simulink model "Simplified_PMSM_Vehicle"  (R2024a)
settings: Solver=ode15s  StartTime=0.0  StopTime=10  RelTol=1e-3  AbsTol=1e-3
undefined symbols (not defined in the file): A, Ca, Ff, Fg, p
libraries: fl_lib x35, nesl_utility x15, ee_lib x3, batteryecm_lib x1
settings Model: Creator=macbookair  LastModifiedBy=macbookair
settings SolverCC: AutoScaleAbsTol=off  AlgebraicLoopSolver=TrustRegion  MaxZcPerStep=1
settings DebuggingCC: UnconnectedInputMsg=warning  UnconnectedOutputMsg=warning  UnconnectedLineMsg=warning  SymbolicDimsDataTypeCodeGenerationDiagnostic=none
settings ModelReferenceCC: EnableRefExpFcnMdlSchedulingChecks=on
settings SFSimCC: CustomCodeUndefinedFunction=UseInterfaceOnly
settings RTWCC: GPUComputeCapability=3.5  DLArmComputeVersion=19.05
settings SimscapeCC: SimscapeLogType=all  SimscapeLogSimulationStatistics=on  SimscapeLogDataHistory=10000

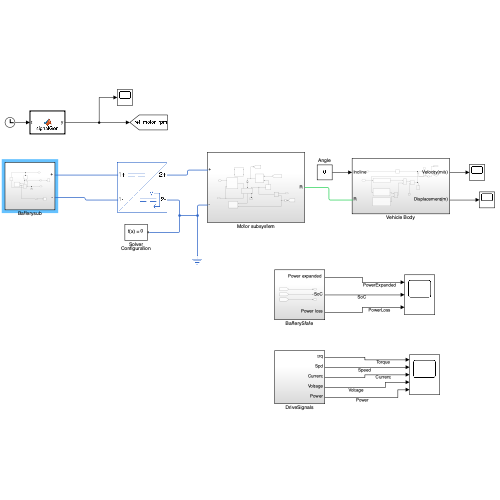
[thumbnail: Simulink's stored preview of the top-level diagram]
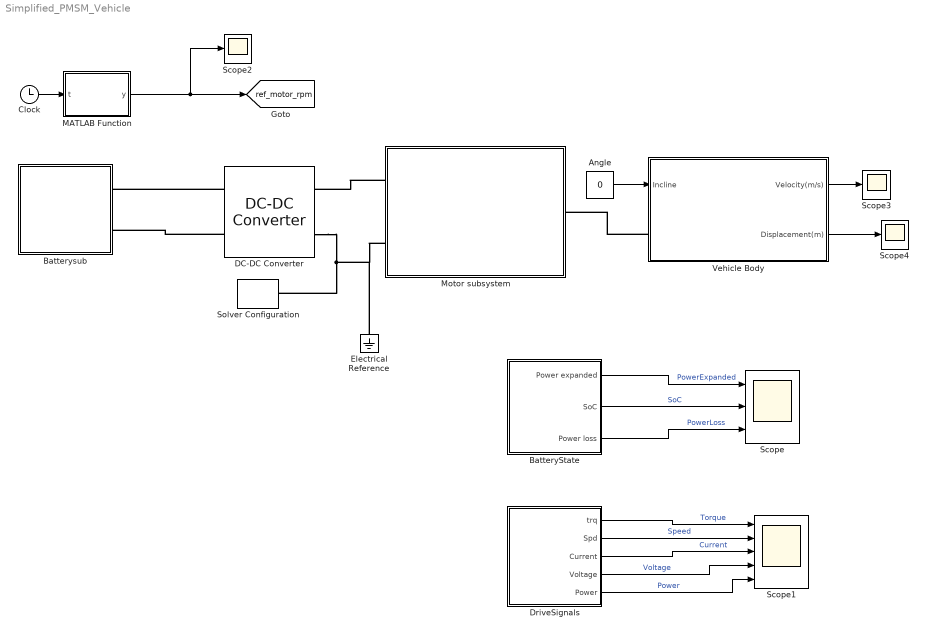
== system Simplified_PMSM_Vehicle ==
  Angle : Constant  Value=0
  BatteryState : Subsystem
  Batterysub : Subsystem
  Clock : Clock
  DC-DC Converter : ee_lib/Semiconductors & Converters/Converters/DC-DC Converter  Vref_option=ee.enum.converters.voltageref.internal  v_ref=500 V  P_rated=200 kW  droop_enabled=true  droop_param=ee.enum.converters.droop.value  droop=0.1 V/A  droop_percent=2  Vref_droop=10 V  reversible=ee.enum.converters.directionality.bidirectional  G_diode=1e-8 1/Ohm  P_fixed=100 W  losses_option=ee.enum.converters.lossesOption.proportionalToSquaredCurrent  eff_rated=97  tableOption=ee.enum.converters.lossTableOptionThermal.currentTemp  i_eff_vec=[-2, -1, 1, 2] A  v_eff_vec=[15, 30, 45] V  eff_vec=[66, 76, 80, 74]  eff_2D_table=[66, 66, 66; 76, 76, 76; 80, 80, 80; 74, 74, 74]  model_dynamics=ee.enum.converters.dynamics.yes  tau=0.02 s  v_ini=500 V  v1_min=1 V  R1=1000 Ohm  R2=1000 Ohm  enable_fault=simscape.enum.onoff.off  fault_condition=ee.enum.faults.faultInputCondition.greaterThan  fault_threshold=0.5  T_eff_vec=[280, 300, 320] K  eff_3D_table=repmat([66; 76; 80; 74], 1, 3, 3)  thermal_mass=100 J/K  initial_temperature=298.15 K
      settings: InternalSimscapePortConfiguration="{\"Bottom\":[],\"Left\":[{\"id\":\"p1\",\"label\":\"1+\",\"type\":\"foundation.electrical.electrical\"},{\"id\":\"n1\",\"label\":\"1-\",\"type\":\"foundation.electrical.electrical\"}],\"Right\":[{\"id\":\"p2\",\"label\":\"2+\",\"type\":\"foundation.electrical.electrical\"},{\"id\":\"n2\",\"label\":\"2-\",\"type\":\"foundation.electrical.electrical\"}],\"Top\":[]}"
  DriveSignals : Subsystem
  Electrical Reference : fl_lib/Electrical/Electrical Elements/Electrical Reference
  MATLAB Function : MATLAB Function  TreatAsAtomicUnit=on
  Motor subsystem : Subsystem
  Scope : Scope  NumInputPorts=3
  Scope1 : Scope  NumInputPorts=5
  Scope2 : Scope
  Scope3 : Scope
  Scope4 : Scope
  Solver Configuration : nesl_utility/Solver Configuration  PhysicalDomain=network_engine_domain  SubClassName=solver  LeftPortType=input  RightPortType=generic  Tones=[]  Harmonics=[]  SimulateNoise=off  Profile=off  UseLocalSampling=off  EnableSwitchedLinearOptims=on  FrequencyDomain=off  UseCCode=off  RelTol=0.001  AbsTol=1e-06  MinStep=1e-09  ToWorkspace=off  RevertToSquareIcSolve=off  NumHomotopyIterations=100  PhasorMode=off  PhasorModeNumHarmonics=1  ConsistencySolver=NEWTON_XTOL_AFTER_FTOL  IndexReductionMethod=DerivativeReplacement  DoDC=off  ResidualTolerance=1e-09  ConsistencyTolSource=GLOBAL  ConsistencyAbsTol=0.001  ConsistencyRelTol=0.001  ConsistencyTolFactor=0.001  UseLocalSolver=off  LocalSolverChoice=NE_BACKWARD_EULER_ADVANCER  ResolveIndetEquations=on  FunctionEvalNumThread=1  LocalSolverSampleTime=0.001  DoFixedCost=off  MaxNonlinIter=3  MaxModeIter=2  ComputeImpulses=off  ImpulseIterations=2  LinearAlgebra=auto  LinearAlgebraNumThread=0  EquationFormulation=NE_TIME_EF  DelaysMemoryBudget=1024  AutomaticFiltering=on  FilteringTimeConstant=0.001  PartitionStorageMethod=AS_NEEDED  PartitionMemoryBudget=1024  PartitionMethod=ROBUST  MultibodyUseLocalSolver=off  MultibodyLocalSolverChoice=ODE1  MultibodyLocalSolverSampleTime=0.001
  Vehicle Body : Subsystem
  tag scope: ref_motor_rpm=global
  wires:
  Clock/1 -> MATLAB Function/1(t)
  Angle/1 -> Vehicle Body/1(Incline)
  BatteryState/1("Power expanded ") -> Scope/1  "PowerExpanded"
  BatteryState/2(SoC) -> Scope/2  "SoC"
  BatteryState/3(Power loss) -> Scope/3  "PowerLoss"
  DriveSignals/1(trq) -> Scope1/1  "Torque"
  DriveSignals/2(Spd) -> Scope1/2  "Speed"
  DriveSignals/3(Current) -> Scope1/3  "Current"
  DriveSignals/4(Voltage) -> Scope1/4  "Voltage"
  DriveSignals/5(Power) -> Scope1/5  "Power"
  MATLAB Function/1(y) -> Scope2/1, [ref_motor_rpm]
  Vehicle Body/1(Velocity(m/s)) -> Scope3/1
  Vehicle Body/2(Displacement(m)) -> Scope4/1
  connections:
  DC-DC Converter/LConn1 -- Batterysub/LConn1
  DC-DC Converter/LConn2 -- Batterysub/LConn2
  DC-DC Converter/RConn2 -- Motor subsystem/LConn2 -- Electrical Reference/LConn1 -- Solver Configuration/RConn1
  Vehicle Body/LConn1 -- Motor subsystem/RConn1
  Motor subsystem/LConn1 -- DC-DC Converter/RConn1

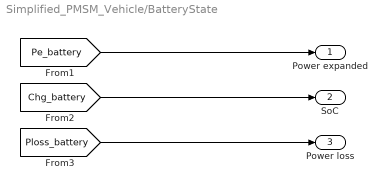
== system Simplified_PMSM_Vehicle/BatteryState ==
  "Power expanded " : Outport
  SoC : Outport  Port=2
  Power loss : Outport  Port=3
  wires:
  [Pe_battery] -> "Power expanded "/1
  [Chg_battery] -> SoC/1
  [Ploss_battery] -> Power loss/1

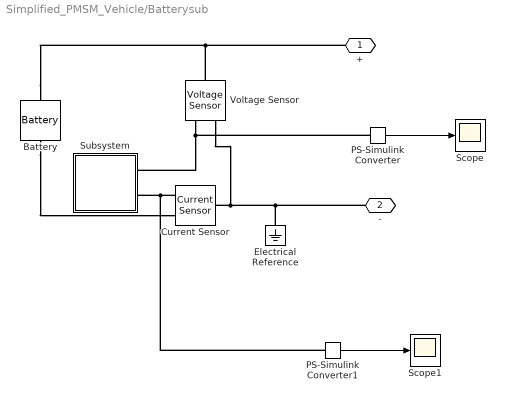
== system Simplified_PMSM_Vehicle/Batterysub ==
  Battery : batteryecm_lib/Battery  Vnom=201.6 V  prm_dir=simscape.enum.battery.prm_dir.disabled  R1_dis=2 Ohm  R1_ch=2 Ohm  R1=0.05 Ohm  prm_AH=simscape.enum.battery.prm_AH.finite  AH=150 A*hr  V1=190 V  AH1=75 A*hr  prm_R2=simscape.enum.battery.prm_R2.disabled  R2=2000 Ohm  Tmeas=298.15 K  charge_measurement_port=simscape.enum.battery.enable.no  prm_dyn=simscape.enum.battery.prm_dyn.off  Rp1=0.005 Ohm  tau1=30 s  Rp2=0.005 Ohm  tau2=30 s  Rp3=0.005 Ohm  tau3=30 s  Rp4=0.005 Ohm  tau4=30 s  Rp5=0.005 Ohm  tau5=30 s  prm_fade=simscape.enum.battery.prm_fade.disabled  N_fade=100  AH_fade=45 A*hr  R1_fade=2.02 Ohm  R1_ch_fade=2.02 Ohm  V1_fade=10.35 V  prm_age=simscape.enum.battery.prm_age.disabled  prm_age_OCV=simscape.enum.battery.prm_age_OCV.OCV  OCV_age=0.9  SOC_age=60  Tmeas_age=298.15 K  delta_time_age_vec=[0] d  temperature_age_vec=[273] K  OCV_scaling_age=2.2134e6  OCV_offset_age=1.632e6  temp_exp_age=0.515833569 V  t_exp_age=0.75  Vnom_T2=12 V  R1_T2=2.2 Ohm  R1_T2_dis=2.2 Ohm  R1_T2_ch=2.2 Ohm  V1_T2=11.4 V  R2_T2=2200 Ohm  Rp1_T2=0.005 Ohm  tau1_T2=30 s  Rp2_T2=0.005 Ohm  tau2_T2=30 s  Rp3_T2=0.005 Ohm  tau3_T2=30 s  Rp4_T2=0.005 Ohm  tau4_T2=30 s  Rp5_T2=0.005 Ohm  tau5_T2=30 s  Tmeas2=273.15 K  thermal_port=simscape.enum.thermaleffects.omit  thermal_mass=30000 J/K  i_specify=off  i_priority=None  i=0 A  i_nominal_specify=off  i_nominal_value=1  i_nominal_unit=A  v_specify=off  v_priority=None  v=0 V  v_nominal_specify=off  v_nominal_value=1  v_nominal_unit=V  charge_specify=on  charge_priority=High  charge=100 A*hr  charge_nominal_specify=off  charge_nominal_value=1  charge_nominal_unit=A*hr  num_cycles_specify=off  num_cycles_priority=High  num_cycles=0  num_cycles_nominal_specify=off  num_cycles_nominal_value=1  num_cycles_nominal_unit=1  temperature_specify=off  temperature_priority=High  temperature=298.15 K  temperature_nominal_specify=off  temperature_nominal_value=1  temperature_nominal_unit=K
  Current Sensor : fl_lib/Electrical/Electrical Sensors/Current Sensor
  Electrical Reference : fl_lib/Electrical/Electrical Elements/Electrical Reference
  PS-Simulink Converter : nesl_utility/PS-Simulink Converter  PhysicalDomain=network_engine_domain  SubClassName=ps_output  LeftPortType=input  RightPortType=output  PseudoPeriodic=off  Frequencies=[]  VectorFormat=inherit  Unit=inherit  AffineConversion=off
  PS-Simulink Converter1 : nesl_utility/PS-Simulink Converter  PhysicalDomain=network_engine_domain  SubClassName=ps_output  LeftPortType=input  RightPortType=output  PseudoPeriodic=off  Frequencies=[]  VectorFormat=inherit  Unit=inherit  AffineConversion=off
  Scope : Scope
  Scope1 : Scope
  Subsystem : Subsystem
  Voltage Sensor : fl_lib/Electrical/Electrical Sensors/Voltage Sensor
  + : PMIOPort  Side=Left
  - : PMIOPort  Port=2  Side=Left
  wires:
  PS-Simulink Converter/1 -> Scope/1
  PS-Simulink Converter1/1 -> Scope1/1
  connections:
  Current Sensor/RConn1 -- PS-Simulink Converter1/LConn1 -- Subsystem/LConn2
  Battery/LConn1 -- +/RConn1 -- Voltage Sensor/LConn1
  Electrical Reference/LConn1 -- -/RConn1 -- Voltage Sensor/RConn2 -- Current Sensor/LConn1
  Voltage Sensor/RConn1 -- Subsystem/LConn1 -- PS-Simulink Converter/LConn1
  Battery/RConn1 -- Current Sensor/RConn2

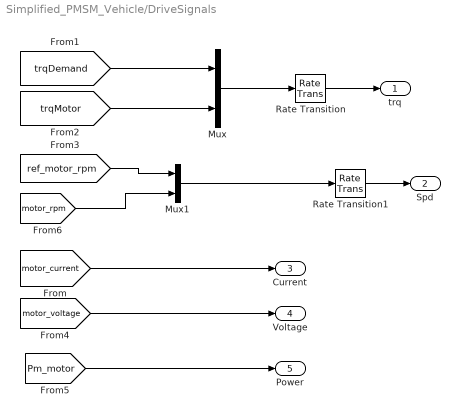
== system Simplified_PMSM_Vehicle/DriveSignals ==
  Mux : Mux  Inputs=2
  Mux1 : Mux  Inputs=2
  Rate Transition : RateTransition
  Rate Transition1 : RateTransition
  trq : Outport
  Spd : Outport  Port=2
  Current : Outport  Port=3
  Voltage : Outport  Port=4
  Power : Outport  Port=5
  wires:
  [trqDemand] -> Mux/1
  [trqMotor] -> Mux/2
  [ref_motor_rpm] -> Mux1/1
  [motor_rpm] -> Mux1/2
  Mux1/1 -> Rate Transition1/1
  Mux/1 -> Rate Transition/1
  [motor_current] -> Current/1
  [motor_voltage] -> Voltage/1
  [Pm_motor] -> Power/1
  Rate Transition/1 -> trq/1
  Rate Transition1/1 -> Spd/1

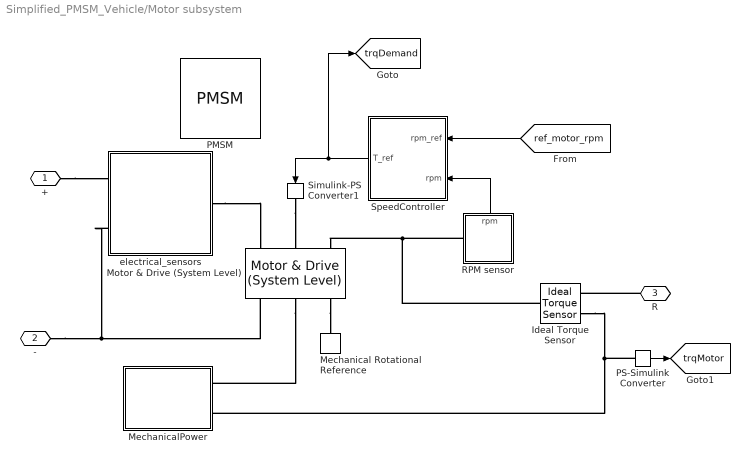
== system Simplified_PMSM_Vehicle/Motor subsystem ==
  Ideal Torque Sensor : fl_lib/Mechanical/Mechanical Sensors/Ideal Torque Sensor
  Mechanical Rotational Reference : fl_lib/Mechanical/Rotational Elements/Mechanical Rotational Reference
  MechanicalPower : Subsystem
  Motor & Drive (System Level) : ee_lib/Electromechanical/Motor & Drive (System Level)  torque_speed_param=ee.enum.electromech.envelope.tabulated  overtorque_param=ee.enum.electromech.overtorque.no  T_t=[.09, .08, .07, 0]*500 N*m  T_t_intermittent=[.36, .32, .28, 0] N*m  T_t_2D=[.09, .09, .09; .08, .08, .08; .07, .07, .07; 0, 0, 0] N*m  T_t_intermittent_2D=[.36, .36, .36; .32, .32, .32; .28, .28, .28; 0, 0, 0] N*m  w_t=[0, 3750, 7500, 8000] rpm  vdc_t=[6, 12, 24] V  torque_max=0.1 N*m  power_max=30 W  torque_max_intermittent=0.4 N*m  power_max_intermittent=120 W  time_overtorque=30 s  time_recover=60 s  Tc=0.02 s  EnableSwitch=false  losses_param=1  eff=95  w_eff=3750 rpm  T_eff=400 N*m  Piron=0 W  Pbase=0 W  w_eff_vec=[-8000, -4000, 0, 4000, 8000] rpm  T_eff_vec=[0, .03, .06, .09] N*m  v_eff_vec=[100, 250, 400] V  losses_mat=[1.49, 1.67, 2.21, 3.1; .42, .69, 1.14, 2.03; .06, .24, .78, 1.68; .42, .69, 1.14, 2.03; 1.49, 1.67, 2.21, 3.1] W  efficiency_mat=[95, 95, 95, 95; 95, 95, 95, 95; 95, 95, 95, 95; 95, 95, 95, 95; 95, 95, 95, 95]  losses_mat_3D=ones(5, 4, 3) W  efficiency_mat_3D=95 * ones(5, 4, 3)  Res=0 Ohm  enable_fault=simscape.enum.onoff.off  fault_condition=1  fault_threshold=0.5  J=0 kg*m^2  lam=1e-5 N*m*s/rad  speed0=0 rpm  faulted_specify=off  faulted_priority=None  faulted=0  faulted_nominal_specify=off  faulted_nominal_value=1  faulted_nominal_unit=1  isSwitchedOff_specify=off  isSwitchedOff_priority=None  isSwitchedOff=0  isSwitchedOff_nominal_specify=off  isSwitchedOff_nominal_value=1  isSwitchedOff_nominal_unit=1  torqueLimitContinuous_specify=off  torqueLimitContinuous_priority=None  torqueLimitContinuous=0 N*m  torqueLimitContinuous_nominal_specify=off  torqueLimitContinuous_nominal_value=1  torqueLimitContinuous_nominal_unit=N*m  alpha=3.93e-3 1/K  Tmeas=25 degC  Tmeas2=125 degC  losses_mat_T2=[1.49, 1.74, 2.49, 3.74; .42, .67, 1.42, 2.67; .06, .31, 1.06, 2.31; .42, .67, 1.42, 2.67; 1.49, 1.74, 2.49, 3.74] W  efficiency_mat_T2=[95, 95, 95, 95; 95, 95, 95, 95; 95, 95, 95, 95; 95, 95, 95, 95; 95, 95, 95, 95]  losses_mat_3D_T2=ones(5, 4, 3) W  efficiency_mat_3D_T2=95 * ones(5, 4, 3)  thermal_mass=100 J/K  initial_temperature=25 degC
  PMSM : ee_lib/Electromechanical/Permanent Magnet/PMSM  port_option=ee.enum.threePhasePort.composite  winding_type=ee.enum.electromech.statorconfiguration.wye  machine_param=ee.enum.pmsm.parameterization.constant  nPolePairs=6  pmflux_param=ee.enum.pmflux.fluxlinkage  pm_flux_linkage=0.03 Wb  torque_constant=0.18 N*m/A  back_emf_constant=0.18 V*s/rad  stator_param=ee.enum.statorparam.LdLqL0  Ld=0.00019 H  Lq=0.00025 H  idVec=[-200, 0, 200] A  iqVec=[-200, 0, 200] A  LdMatrix=0.0002 * ones(3, 3) H  LqMatrix=0.0002 * ones(3, 3) H  PmMatrix=0.1 * ones(3, 3) Wb  ktMatrix=0.18 * ones(3, 3) N*m/A  keMatrix=0.18 * ones(3, 3) V*s/rad  L0=0.00016 H  Ls=0.0002 H  Lm=-0.00002 H  Ms=0.00002 H  Rs=0.013 Ohm  zero_sequence=ee.enum.park.zerosequence.include  axes_param=ee.enum.rotorangle.daxis  loss_param=ee.enum.ironloss.none  losses_oc=[0, 0, 0] W  losses_sc=[0, 0, 0] W  f_losses=60 Hz  Isc_losses=95 A  J=0.01 kg*m^2  lam=0 N*m*s/rad  i_d_specify=off  i_d_priority=None  i_d=0 A  i_d_nominal_specify=off  i_d_nominal_value=1  i_d_nominal_unit=A  i_q_specify=off  i_q_priority=None  i_q=0 A  i_q_nominal_specify=off  i_q_nominal_value=1  i_q_nominal_unit=A  torque_specify=off  torque_priority=None  torque=0 N*m  torque_nominal_specify=off  torque_nominal_value=1  torque_nominal_unit=N*m  angular_velocity_specify=off  angular_velocity_priority=High  angular_velocity=0 rpm  angular_velocity_nominal_specify=off  angular_velocity_nominal_value=1  angular_velocity_nominal_unit=rpm  angular_position_specify=off  angular_position_priority=High  angular_position=0 deg  angular_position_nominal_specify=off  angular_position_nominal_value=1  angular_position_nominal_unit=deg  alpha=3.93e-3 1/K  alpha_flux=-0.001 1/K  Tmeas=298.15 K  stator_thermal_mass=100 J/K  rotor_thermal_mass=200 J/K  Rm_percent_rotor=90  Rd_percent_rotor=30  temperatureA_specify=off  temperatureA_priority=High  temperatureA=25 degC  temperatureA_nominal_specify=off  temperatureA_nominal_value=1  temperatureA_nominal_unit=degC  temperatureB_specify=off  temperatureB_priority=High  temperatureB=25 degC  temperatureB_nominal_specify=off  temperatureB_nominal_value=1  temperatureB_nominal_unit=degC  temperatureC_specify=off  temperatureC_priority=High  temperatureC=25 degC  temperatureC_nominal_specify=off  temperatureC_nominal_value=1  temperatureC_nominal_unit=degC  temperatureR_specify=off  temperatureR_priority=High  temperatureR=25 degC  temperatureR_nominal_specify=off  temperatureR_nominal_value=1  temperatureR_nominal_unit=degC
      settings: InternalSimscapePortConfiguration="{\"Bottom\":[],\"Left\":[{\"id\":\"N\",\"label\":\"~\",\"type\":\"foundation.electrical.three_phase\"},{\"id\":\"n\",\"label\":\"n\",\"type\":\"foundation.electrical.electrical\"}],\"Right\":[{\"id\":\"R\",\"label\":\"R\",\"type\":\"foundation.mechanical.rotational.rotational\"},{\"id\":\"C\",\"label\":\"C\",\"type\":\"foundation.mechanical.rotational.rotational\"}],\"Top\":[]}"
  PS-Simulink Converter : nesl_utility/PS-Simulink Converter  PhysicalDomain=network_engine_domain  SubClassName=ps_output  LeftPortType=input  RightPortType=output  PseudoPeriodic=off  Frequencies=[]  VectorFormat=inherit  Unit=N*m  AffineConversion=off
  RPM sensor : Subsystem
      settings: PortSchema="{\"entries\":[{\"content\":{\"sides\":[{\"content\":{\"connectorIds\":[\"LConn1\"]},\"type\":\"ConnectorPlacement.EquallySpacedRectSide\",\"uuid\":\"39d046d5-f421-4f0d-879d-c19748025329\"},{\"content\":{\"side\":\"RIGHT\"},\"type\":\"ConnectorPlacement.EquallySpacedRectSide\",\"uuid\":\"b6149d9e-7ab3-4f68-a15b-9fef8f2169c7\"},{\"content\":{\"connectorIds\":[\"Out1\"],\"side\":\"TOP\"},\"type\":\"ConnectorPlacement.EquallySpacedRectSide\",\"uuid\":\"8d72c58d-98ea-41b6-b92c-6f7faea464b9\"}]},\"type\":\"ConnectorPlacement.EquallySpacedConnector\",\"uuid\":\"adc7404a-30c2-4f0e-88a4-d697cd090ad2\"}],\"packageUris\":[\"http://schema.mathworks.com/mf0/Connector/R2020b\"],\"version\":\"1.0\"}"
  Simulink-PS Converter1 : nesl_utility/Simulink-PS Converter  PhysicalDomain=network_engine_domain  SubClassName=ps_input  LeftPortType=input  RightPortType=output  PseudoPeriodic=off  Frequencies=[]  NoiseDistribution=none  NoiseParameters=[]  Unit=N*m  AffineConversion=off  FilteringAndDerivatives=provide  SimscapeFilterOrder=1  InputFilterTimeConstant=0.001  UdotUserProvided=0
  SpeedController : Subsystem
  electrical_sensors : Subsystem
  + : PMIOPort  Side=Left
  - : PMIOPort  Port=2  Side=Left
  R : PMIOPort  Port=3  Side=Right
  tag scope: trqDemand=global, trqMotor=global
  wires:
  PS-Simulink Converter/1 -> [trqMotor]
  SpeedController/1(T_ref) -> [trqDemand], Simulink-PS Converter1/1
  RPM sensor/1(rpm) -> SpeedController/2(rpm)
  [ref_motor_rpm] -> SpeedController/1(rpm_ref)
  connections:
  Simulink-PS Converter1/RConn1 -- Motor & Drive (System Level)/LConn2
  Motor & Drive (System Level)/RConn1 -- -/RConn1 -- electrical_sensors/LConn2
  R/RConn1 -- Ideal Torque Sensor/RConn1
  Motor & Drive (System Level)/RConn3 -- Mechanical Rotational Reference/LConn1
  RPM sensor/LConn1 -- Ideal Torque Sensor/LConn1 -- Motor & Drive (System Level)/LConn3
  electrical_sensors/RConn1 -- Motor & Drive (System Level)/LConn1
  Motor & Drive (System Level)/RConn2 -- MechanicalPower/LConn1
  Ideal Torque Sensor/RConn2 -- PS-Simulink Converter/LConn1 -- MechanicalPower/LConn2
  +/RConn1 -- electrical_sensors/LConn1

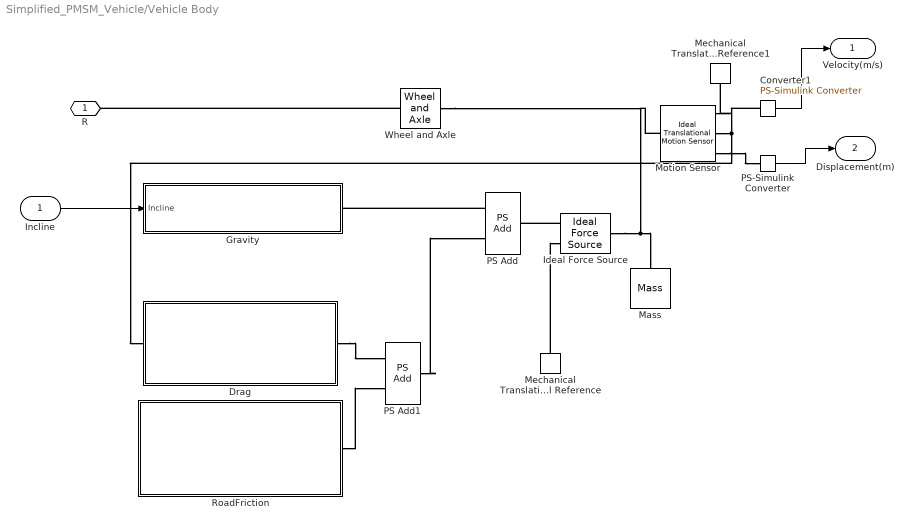
== system Simplified_PMSM_Vehicle/Vehicle Body ==
  Incline : Inport
  Converter1 : nesl_utility/PS-Simulink Converter  PhysicalDomain=network_engine_domain  SubClassName=ps_output  LeftPortType=input  RightPortType=output  PseudoPeriodic=off  Frequencies=[]  VectorFormat=inherit  Unit=m/s  AffineConversion=off
  Drag : Subsystem
  Gravity : Subsystem
  Ideal Force Source : fl_lib/Mechanical/Mechanical Sources/Ideal Force Source
  Mass : fl_lib/Mechanical/Translational Elements/Mass  mass=Mv kg  num_ports=foundation.enum.numPorts2.one  v_specify=off  v_priority=High  v=0 m/s  v_nominal_specify=off  v_nominal_value=1  v_nominal_unit=m/s  f_specify=off  f_priority=None  f=0 N  f_nominal_specify=off  f_nominal_value=1  f_nominal_unit=N
  Mechanical Translational Reference : fl_lib/Mechanical/Translational Elements/Mechanical Translational Reference
  Mechanical Translational Reference1 : fl_lib/Mechanical/Translational Elements/Mechanical Translational Reference
  Motion Sensor : fl_lib/Mechanical/Mechanical Sensors/Ideal Translational Motion Sensor  reference=foundation.enum.MeasurementReference.difference  acceleration_port=false  velocity_port=true  position_port=true  offset=0 m
  PS Add : fl_lib/Physical Signals/Functions/PS Add
  PS Add1 : fl_lib/Physical Signals/Functions/PS Add
  PS-Simulink Converter : nesl_utility/PS-Simulink Converter  PhysicalDomain=network_engine_domain  SubClassName=ps_output  LeftPortType=input  RightPortType=output  PseudoPeriodic=off  Frequencies=[]  VectorFormat=inherit  Unit=m  AffineConversion=off
  RoadFriction : Subsystem
  Wheel and Axle : fl_lib/Mechanical/Mechanisms/Wheel and Axle  R=0.3 m  or=1  t_specify=off  t_priority=None  t=0 N*m  t_nominal_specify=off  t_nominal_value=1  t_nominal_unit=N*m  f_specify=off  f_priority=None  f=0 N  f_nominal_specify=off  f_nominal_value=1  f_nominal_unit=N
  R : PMIOPort  Side=Left
  Velocity(m/s) : Outport
  Displacement(m) : Outport  Port=2
  wires:
  Converter1/1 -> Velocity(m/s)/1
  Incline/1 -> Gravity/1(Incline)
  PS-Simulink Converter/1 -> Displacement(m)/1
  connections:
  PS Add1/RConn1 -- PS Add/LConn2
  Ideal Force Source/LConn1 -- Wheel and Axle/RConn1 -- Motion Sensor/LConn1 -- Mass/LConn1
  Motion Sensor/RConn2 -- Drag/LConn1 -- Converter1/LConn1
  Ideal Force Source/RConn1 -- PS Add/RConn1
  Mechanical Translational Reference/LConn1 -- Ideal Force Source/RConn2
  PS Add/LConn1 -- Gravity/RConn1
  Drag/RConn1 -- PS Add1/LConn1
  RoadFriction/RConn1 -- PS Add1/LConn2
  Motion Sensor/RConn3 -- PS-Simulink Converter/LConn1
  Motion Sensor/RConn1 -- Mechanical Translational Reference1/LConn1
  Wheel and Axle/LConn1 -- R/RConn1

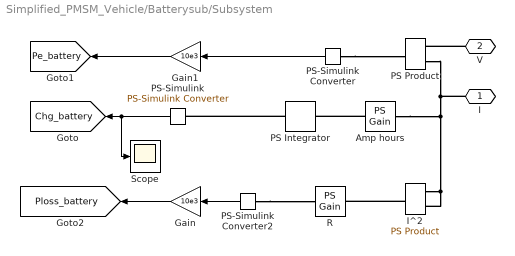
== system Simplified_PMSM_Vehicle/Batterysub/Subsystem ==
  Amp hours : fl_lib/Physical Signals/Functions/PS Gain  gain=5/3600
  Gain : Gain  Gain=10e3
  Gain1 : Gain  Gain=10e3
  I^2 : fl_lib/Physical Signals/Functions/PS Product
  PS Integrator : fl_lib/Physical Signals/Linear Operators/PS Integrator  reset_method=foundation.enum.IntegratorResetSpec.None  initial_condition_spec=foundation.enum.IntegratorICSpec.Internal  saturation_spec=foundation.enum.IntegratorSaturationSpec.None  saturation_source_spec=foundation.enum.IntegratorSaturationSourceSpec.Internal  x0=0 s  xu=inf s  xl=-inf s
  PS Product : fl_lib/Physical Signals/Functions/PS Product
  "PS-Simulink " : nesl_utility/PS-Simulink Converter  PhysicalDomain=network_engine_domain  SubClassName=ps_output  LeftPortType=input  RightPortType=output  PseudoPeriodic=off  Frequencies=[]  VectorFormat=inherit  Unit=inherit  AffineConversion=off
  PS-Simulink Converter : nesl_utility/PS-Simulink Converter  PhysicalDomain=network_engine_domain  SubClassName=ps_output  LeftPortType=input  RightPortType=output  PseudoPeriodic=off  Frequencies=[]  VectorFormat=inherit  Unit=inherit  AffineConversion=off
  PS-Simulink Converter2 : nesl_utility/PS-Simulink Converter  PhysicalDomain=network_engine_domain  SubClassName=ps_output  LeftPortType=input  RightPortType=output  PseudoPeriodic=off  Frequencies=[]  VectorFormat=inherit  Unit=inherit  AffineConversion=off
  R : fl_lib/Physical Signals/Functions/PS Gain  gain=1
  Scope : Scope
  I : PMIOPort  Side=Left
  V : PMIOPort  Port=2  Side=Left
  tag scope: Chg_battery=global, Pe_battery=global, Ploss_battery=global
  wires:
  PS-Simulink Converter2/1 -> Gain/1
  Gain/1 -> [Ploss_battery]
  PS-Simulink Converter/1 -> Gain1/1
  Gain1/1 -> [Pe_battery]
  "PS-Simulink "/1 -> Scope/1, [Chg_battery]
  connections:
  PS Product/LConn2 -- I/RConn1 -- I^2/LConn1 -- I^2/LConn2 -- Amp hours/LConn1
  PS-Simulink Converter2/LConn1 -- R/RConn1
  PS-Simulink Converter/LConn1 -- PS Product/RConn1
  I^2/RConn1 -- R/LConn1
  Amp hours/RConn1 -- PS Integrator/LConn1
  V/RConn1 -- PS Product/LConn1
  PS Integrator/RConn1 -- "PS-Simulink "/LConn1

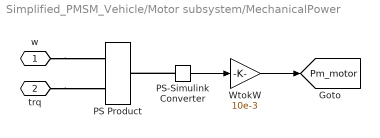
== system Simplified_PMSM_Vehicle/Motor subsystem/MechanicalPower ==
  PS Product : fl_lib/Physical Signals/Functions/PS Product
  PS-Simulink Converter : nesl_utility/PS-Simulink Converter  PhysicalDomain=network_engine_domain  SubClassName=ps_output  LeftPortType=input  RightPortType=output  PseudoPeriodic=off  Frequencies=[]  VectorFormat=inherit  Unit=inherit  AffineConversion=off
  WtokW : Gain  Gain=10e-3
  w : PMIOPort  Side=Left
  trq : PMIOPort  Port=2  Side=Left
  tag scope: Pm_motor=global
  wires:
  PS-Simulink Converter/1 -> WtokW/1
  WtokW/1 -> [Pm_motor]
  connections:
  trq/RConn1 -- PS Product/LConn2
  w/RConn1 -- PS Product/LConn1
  PS-Simulink Converter/LConn1 -- PS Product/RConn1

== system Simplified_PMSM_Vehicle/Motor subsystem/RPM sensor ==
  Ideal Rotational Motion Sensor : fl_lib/Mechanical/Mechanical Sensors/Ideal Rotational Motion Sensor  reference=foundation.enum.MeasurementReference.difference  acceleration_port=false  velocity_port=true  position_port=true  wrap_angle=false  offset=0 rad
  Mechanical Rotational Reference : fl_lib/Mechanical/Rotational Elements/Mechanical Rotational Reference
  PS-Simulink Converter : nesl_utility/PS-Simulink Converter  PhysicalDomain=network_engine_domain  SubClassName=ps_output  LeftPortType=input  RightPortType=output  PseudoPeriodic=off  Frequencies=[]  VectorFormat=inherit  Unit=inherit  AffineConversion=off
  R : PMIOPort  Side=Left
  rpm : Outport
  tag scope: motor_rpm=global
  wires:
  PS-Simulink Converter/1 -> [motor_rpm], rpm/1
  connections:
  Mechanical Rotational Reference/LConn1 -- Ideal Rotational Motion Sensor/RConn1
  Ideal Rotational Motion Sensor/RConn2 -- PS-Simulink Converter/LConn1
  R/RConn1 -- Ideal Rotational Motion Sensor/LConn1

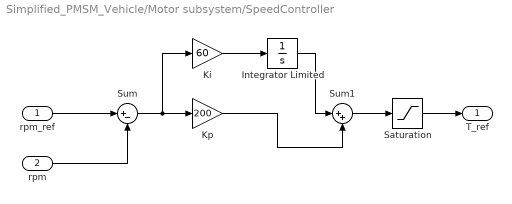
== system Simplified_PMSM_Vehicle/Motor subsystem/SpeedController ==
  rpm_ref : Inport
  rpm : Inport  Port=2
  Integrator Limited : Integrator  LimitOutput=on  UpperSaturationLimit=40  LowerSaturationLimit=-40
  Ki : Gain  Gain=60
  Kp : Gain  Gain=200
  Saturation : Saturate  UpperLimit=400  LowerLimit=-40
  Sum : Sum  Inputs=|+-
  Sum1 : Sum  Inputs=|++
  T_ref : Outport
  wires:
  rpm_ref/1 -> Sum/1
  rpm/1 -> Sum/2
  Sum/1 -> Ki/1, Kp/1
  Ki/1 -> Integrator Limited/1
  Kp/1 -> Sum1/2
  Integrator Limited/1 -> Sum1/1
  Sum1/1 -> Saturation/1
  Saturation/1 -> T_ref/1

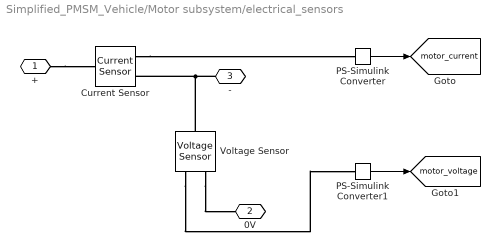
== system Simplified_PMSM_Vehicle/Motor subsystem/electrical_sensors ==
  Current Sensor : fl_lib/Electrical/Electrical Sensors/Current Sensor
  PS-Simulink Converter : nesl_utility/PS-Simulink Converter  PhysicalDomain=network_engine_domain  SubClassName=ps_output  LeftPortType=input  RightPortType=output  PseudoPeriodic=off  Frequencies=[]  VectorFormat=inherit  Unit=inherit  AffineConversion=off
  PS-Simulink Converter1 : nesl_utility/PS-Simulink Converter  PhysicalDomain=network_engine_domain  SubClassName=ps_output  LeftPortType=input  RightPortType=output  PseudoPeriodic=off  Frequencies=[]  VectorFormat=inherit  Unit=inherit  AffineConversion=off
  Voltage Sensor : fl_lib/Electrical/Electrical Sensors/Voltage Sensor
  + : PMIOPort  Side=Left
  0V : PMIOPort  Port=2  Side=Left
  - : PMIOPort  Port=3  Side=Right
  tag scope: motor_current=global, motor_voltage=global
  wires:
  PS-Simulink Converter/1 -> [motor_current]
  PS-Simulink Converter1/1 -> [motor_voltage]
  connections:
  +/RConn1 -- Current Sensor/LConn1
  -/RConn1 -- Current Sensor/RConn2 -- Voltage Sensor/LConn1
  Voltage Sensor/RConn2 -- 0V/RConn1
  Voltage Sensor/RConn1 -- PS-Simulink Converter1/LConn1
  Current Sensor/RConn1 -- PS-Simulink Converter/LConn1

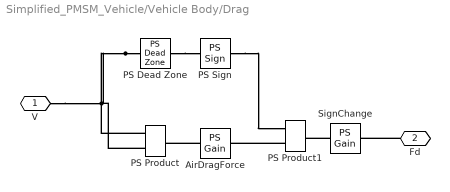
== system Simplified_PMSM_Vehicle/Vehicle Body/Drag ==
  AirDragForce : fl_lib/Physical Signals/Functions/PS Gain  gain=0.5 * Ca * A * p
  PS Dead Zone : fl_lib/Physical Signals/Nonlinear Operators/PS Dead Zone  upper_limit=0.5 m/s  lower_limit=-0.5 m/s
      settings: InternalSimscapePortConfiguration="{\"Bottom\":[],\"Left\":[{\"id\":\"I\",\"label\":\"\",\"type\":\"input\"}],\"Right\":[{\"id\":\"O\",\"label\":\"\",\"type\":\"output\"}],\"Top\":[]}"
  PS Product : fl_lib/Physical Signals/Functions/PS Product
  PS Product1 : fl_lib/Physical Signals/Functions/PS Product
  PS Sign : fl_lib/Physical Signals/Nonlinear Operators/PS Sign
      settings: InternalSimscapePortConfiguration="{\"Bottom\":[],\"Left\":[{\"id\":\"I\",\"label\":\"\",\"type\":\"input\"}],\"Right\":[{\"id\":\"O\",\"label\":\"\",\"type\":\"output\"}],\"Top\":[]}"
  SignChange : fl_lib/Physical Signals/Functions/PS Gain  gain=-1 N*(s^2/m^2)
  V : PMIOPort  Side=Left
  Fd : PMIOPort  Port=2  Side=Right
  connections:
  PS Dead Zone/RConn1 -- PS Sign/LConn1
  AirDragForce/LConn1 -- PS Product/RConn1
  PS Sign/RConn1 -- PS Product1/LConn1
  PS Product1/LConn2 -- AirDragForce/RConn1
  SignChange/LConn1 -- PS Product1/RConn1
  PS Dead Zone/LConn1 -- V/RConn1 -- PS Product/LConn2 -- PS Product/LConn1
  Fd/RConn1 -- SignChange/RConn1

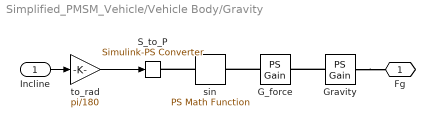
== system Simplified_PMSM_Vehicle/Vehicle Body/Gravity ==
  Incline : Inport
  G_force : fl_lib/Physical Signals/Functions/PS Gain  gain=Fg N
  Gravity : fl_lib/Physical Signals/Functions/PS Gain  gain=-1
  S_to_P : nesl_utility/Simulink-PS Converter  PhysicalDomain=network_engine_domain  SubClassName=ps_input  LeftPortType=input  RightPortType=output  PseudoPeriodic=off  Frequencies=[]  NoiseDistribution=none  NoiseParameters=[]  Unit=1  AffineConversion=off  FilteringAndDerivatives=provide  SimscapeFilterOrder=1  InputFilterTimeConstant=0.001  UdotUserProvided=0
  sin : fl_lib/Physical Signals/Functions/PS Math Function  fcn_choice=foundation.enum.math_function.sin  v=1
  to_rad : Gain  Gain=pi/180
  Fg : PMIOPort  Side=Right
  wires:
  Incline/1 -> to_rad/1
  to_rad/1 -> S_to_P/1
  connections:
  sin/LConn1 -- S_to_P/RConn1
  G_force/LConn1 -- sin/RConn1
  Gravity/RConn1 -- Fg/RConn1
  Gravity/LConn1 -- G_force/RConn1

== system Simplified_PMSM_Vehicle/Vehicle Body/RoadFriction ==
  PS Gain : fl_lib/Physical Signals/Functions/PS Gain  gain=Ff N
  frictionForce : fl_lib/Physical Signals/Functions/PS Gain  gain=-1
  Ff : PMIOPort  Side=Right
  connections:
  frictionForce/RConn1 -- Ff/RConn1
  frictionForce/LConn1 -- PS Gain/RConn1

== matlab function Simplified_PMSM_Vehicle/MATLAB Function ==
  data: t input; y output
function y = signalGen(t)
if t < 0
    y = 0;
elseif t >= 0 && t < 4
    y = (100 / 4) * t;
elseif t >= 4 && t < 6
    y = 100;
elseif t >= 6 && t <= 11
    y = 100 - ((100 / 4) * (t - 6));
else
    y = 0;
end
